simulink model "BD_PAR_SS"  (Simulink 10.3)
settings: Solver=ode1  StartTime=0.0  StopTime=max(cyc_mph(:,1))  FixedStep=1  MaxStep=1  RelTol=1e-3  AbsTol=1e-3
undefined symbols (not defined in the file): acc_elec_eff, acc_elec_pwr, acc_mech_eff, amb_tmp, cs_charge_deplete_bool, cs_electric_decel_spd, cs_electric_launch_spd_hi, cs_electric_launch_spd_lo, cs_hi_soc, cs_lo_soc, cs_off_trq_frac, cyc_avg_time, cyc_cargo_mass, cyc_elevation_init, cyc_filter_bool, cyc_grade, cyc_mph, ess_module_num, ess_on, ess_voc, ex_calc, ex_cat_co_frac, ex_cat_ext_cp, ex_cat_ext_emisv, ex_cat_ext_init_tmp, ex_cat_ext_mass, ex_cat_ext_sarea, ex_cat_hc_frac, ex_cat_i2p_th_cond, ex_cat_i2x_emisv, ex_cat_i2x_th_cond, ex_cat_int_cp, ex_cat_int_init_tmp, ex_cat_int_mass, ex_cat_int_sarea, ex_cat_lim, ex_cat_m2i_th_cond, ex_cat_m2i_tmp, ex_cat_m2p_emisv, ex_cat_mon_cp, ex_cat_mon_init_tmp, ex_cat_mon_mass, ex_cat_mon_sarea, ex_cat_monf_sarea, ex_cat_moni_sarea, ex_cat_nox_frac, ex_cat_p2x_th_cond, ex_cat_pcm_ecp, ex_cat_pcm_mass, ex_cat_pcm_tmp, ex_cat_pipe_cp, ex_cat_pipe_emisv, ex_cat_pipe_init_tmp, ex_cat_pipe_mass, ex_cat_pipe_sarea, ex_cat_pm_frac, ex_cat_tmp_range, ex_gas_cp, ex_manif_cp, ex_manif_emisv ... (+73)
libraries: lib_controls x6, lib_vehicle x3, lib_accessory x2, lib_interactive x1, lib_energy_storage x1, lib_fuel_converter x1
(part 5 of 6)

== system BD_PAR_SS/exhaust sys <ex>/ex gas heat flow/Block NOTES ==
  note: EXHAUST GAS HEAT TRANSFER
      | This block models the heat loss from the exhaust gas as it flows from the engine through the manifold,
      | downpipe, and catalytic converter.  Also included is the increase in gas temperature within the converter
      | due to the catalysis of HC, CO, and NOx. The block is conditionally executed only if engine_on=1.

== system BD_PAR_SS/exhaust sys <ex>/ex gas heat flow/converter ==
  h,exg : Inport
  Cexg : Inport  Port=2
  Texgi : Inport  Port=3
  Tex : Inport  Port=4
  " Q/C" : Product  Inputs=/*  SaturateOnIntegerOverflow=on
  1/A : Gain  Gain=1/(ex_cat_moni_sarea+ex_cat_int_sarea-ex_cat_mon_sarea)  SaturateOnIntegerOverflow=on
  Demux3 : Demux  Outputs=2
  MinMax : MinMax  Inputs=2
  Mux16 : Mux
  Qci2g_ : Fcn  Expr=u(1)*(ex_cat_int_sarea - ex_cat_mon_sarea)*(u(3)-u(4))
  Qcm2g_ : Fcn  Expr=u(1)*ex_cat_moni_sarea*(u(2)-u(4))
  Selector3 : Selector  InputPortWidth=5  IndexOptions=Index vector (dialog)  Indices=[ 1 2 ]  OutputSizes=1
  T : Sum  SaturateOnIntegerOverflow=on
  T1 : Sum  SaturateOnIntegerOverflow=on
  Texgo : Outport  OutputWhenDisabled=reset  InitialOutput=amb_tmp
  Qcm2g : Outport  Port=2  OutputWhenDisabled=reset  InitialOutput=0
  Qci2g : Outport  Port=3  OutputWhenDisabled=reset  InitialOutput=0
  wires:
  Cexg/1 -> " Q/C"/1, 1/A/1
  h,exg/1 -> MinMax/2
  1/A/1 -> MinMax/1
  MinMax/1 -> Mux16/1
  Tex/1 -> Selector3/1
  Selector3/1 -> Demux3/1
  Demux3/1 -> Mux16/2
  Demux3/2 -> Mux16/3
  Texgi/1 -> T/2, Mux16/4
  Mux16/1 -> Qcm2g_/1, Qci2g_/1
  Qci2g_/1 -> T1/2, Qci2g/1
  Qcm2g_/1 -> T1/1, Qcm2g/1
  " Q/C"/1 -> T/1
  T1/1 -> " Q/C"/2
  T/1 -> Texgo/1

== system BD_PAR_SS/exhaust sys <ex>/ex gas heat flow/inlet pipe ==
  h,exg : Inport
  Cexg : Inport  Port=2
  Texgi : Inport  Port=3
  Tex : Inport  Port=4
  " Q/C" : Product  Inputs=/*  SaturateOnIntegerOverflow=on
  A : Gain  Gain=ex_cat_pipe_sarea  SaturateOnIntegerOverflow=on
  Memory : Memory  InitialCondition=cyc_mph(1,2)*.447
  MinMax : MinMax  Inputs=2
  Mux19 : Mux  Inputs=3
  Selector2 : Selector  InputPortWidth=5  IndexOptions=Index vector (dialog)  Indices=3  OutputSizes=1
  T : Sum  SaturateOnIntegerOverflow=on
  Ts-Tex,ave : Fcn  Expr=u(2) - (u(3)+u(1))/2
  tailpipe  emis : Product  SaturateOnIntegerOverflow=on
  Texgo : Outport  OutputWhenDisabled=reset  InitialOutput=amb_tmp
  tag scope: Qp2g=global, Tgpo=global
  wires:
  h,exg/1 -> A/1
  MinMax/1 -> tailpipe  emis/1
  A/1 -> MinMax/2
  Cexg/1 -> MinMax/1, " Q/C"/1
  tailpipe  emis/1 -> " Q/C"/2, [Qp2g]
  " Q/C"/1 -> T/1
  Texgi/1 -> T/2, Mux19/1
  T/1 -> Texgo/1, [Tgpo], Memory/1
  Tex/1 -> Selector2/1
  Mux19/1 -> Ts-Tex,ave/1
  Ts-Tex,ave/1 -> tailpipe  emis/2
  Selector2/1 -> Mux19/2
  Memory/1 -> Mux19/3

== system BD_PAR_SS/exhaust sys <ex>/ex gas heat flow/manifold  ==
  h,exg : Inport
  Cexg : Inport  Port=2
  Texgi : Inport  Port=3
  Tex : Inport  Port=4
  " Q/C" : Product  Inputs=/*  SaturateOnIntegerOverflow=on
  A : Gain  Gain=ex_manif_sarea  SaturateOnIntegerOverflow=on
  Memory : Memory  InitialCondition=cyc_mph(1,2)*.447
  MinMax : MinMax  Inputs=2
  Mux19 : Mux  Inputs=3
  Selector1 : Selector  InputPortWidth=5  IndexOptions=Index vector (dialog)  Indices=5  OutputSizes=1
  T : Sum  SaturateOnIntegerOverflow=on
  Ts-Tex,ave : Fcn  Expr=u(2) - (u(3)+u(1))/2
  tailpipe  emis : Product  SaturateOnIntegerOverflow=on
  Texgo : Outport  OutputWhenDisabled=reset  InitialOutput=amb_tmp
  tag scope: Qma2g=global, Tgmo=global
  wires:
  h,exg/1 -> A/1
  MinMax/1 -> tailpipe  emis/1
  A/1 -> MinMax/2
  Cexg/1 -> MinMax/1, " Q/C"/1
  " Q/C"/1 -> T/1
  T/1 -> [Tgmo], Texgo/1, Memory/1
  tailpipe  emis/1 -> " Q/C"/2, [Qma2g]
  Tex/1 -> Selector1/1
  Selector1/1 -> Mux19/2
  Mux19/1 -> Ts-Tex,ave/1
  Memory/1 -> Mux19/3
  Ts-Tex,ave/1 -> tailpipe  emis/2
  Texgi/1 -> Mux19/1, T/2

== system BD_PAR_SS/exhaust sys <ex>/ex sys heat flow/Block NOTES ==
  note: CATALYTIC CONVERTER HEAT LOSS
      | This block models the heat loss from a catalytic converter (conventional or vacuum-insulated).
      | Convection (as a function of vehicle speed), radiation, and conduction effects are included.
      | Converter monolith (m), interior (i), pipe (p), and exterior (x) and engine manifold
      | heat flows are estimated based on the temperatures from the previous iteration.

== system BD_PAR_SS/exhaust sys <ex>/removal efficiencies/removal efficiencies (base ADVISOR) ==
  Ex Cat T (C) : Inport
  Enable : EnablePort  StatesWhenEnabling=reset
  CO temp eff : Lookup  InputValues=ex_cat_tmp_range  Table=ex_cat_co_frac  SaturateOnIntegerOverflow=on
  HC temp eff : Lookup  InputValues=ex_cat_tmp_range  Table=ex_cat_hc_frac  SaturateOnIntegerOverflow=on
  Mux : Mux
  NOx temp eff : Lookup  InputValues=ex_cat_tmp_range  Table=ex_cat_nox_frac  SaturateOnIntegerOverflow=on
  PM temp eff : Lookup  InputValues=ex_cat_tmp_range  Table=ex_cat_pm_frac  SaturateOnIntegerOverflow=on
  removal effs : Outport  OutputWhenDisabled=reset  InitialOutput=0
  wires:
  Ex Cat T (C)/1 -> PM temp eff/1, NOx temp eff/1, CO temp eff/1, HC temp eff/1
  Mux/1 -> removal effs/1
  PM temp eff/1 -> Mux/4
  NOx temp eff/1 -> Mux/3
  HC temp eff/1 -> Mux/1
  CO temp eff/1 -> Mux/2

== system BD_PAR_SS/exhaust sys <ex>/removal efficiencies/removal efficiencies ORNL ==
  gas_flow (g/s) : Inport
  Ex Gas T (C) : Inport  Port=2
  O2_exh (g/s) : Inport  Port=3
  emis Engine Out (g/s) : Inport  Port=4
  Ex Cat T (C) : Inport  Port=5
  Enable : EnablePort  StatesWhenEnabling=reset
  CO : Terminator
  CO-Conversion : Subsystem
  Constant : Constant  Value=1200
  Demux : Demux
  HC-Conversion : Subsystem
  Mux : Mux
  NOx_Eff : Subsystem
  PM : Terminator
  PM temp eff : Lookup  InputValues=ex_cat_tmp_range  Table=ex_cat_pm_frac  SaturateOnIntegerOverflow=on
  Product : Product  Inputs=/*  SaturateOnIntegerOverflow=on
  Volume  Flow (m^3/sec) : Gain  Gain=2.96E6  SaturateOnIntegerOverflow=on
  removal effs : Outport  OutputWhenDisabled=reset  InitialOutput=0
  wires:
  Mux/1 -> removal effs/1
  gas_flow (g/s)/1 -> CO-Conversion/4(ex_gas_flow), HC-Conversion/4(ex_gas_flow), Product/2
  Ex Cat T (C)/1 -> PM temp eff/1
  O2_exh (g/s)/1 -> CO-Conversion/3(O2_exh), HC-Conversion/3(O2_exh)
  CO-Conversion/1(CO_eff) -> Mux/2
  HC-Conversion/1(HC_eff) -> Mux/1
  NOx_Eff/1(NOx_eff) -> Mux/3
  PM temp eff/1 -> Mux/4
  Ex Gas T (C)/1 -> NOx_Eff/2(Ex_temp), CO-Conversion/2(T_exh), HC-Conversion/2(T_exh)
  Volume  Flow (m^3/sec)/1 -> NOx_Eff/1(vol_flow), CO-Conversion/1(vol_flow), HC-Conversion/1(vol_flow)
  Demux/1 -> NOx_Eff/3(HC_Inlet)
  Demux/3 -> NOx_Eff/4(NOx_Inlet)
  Demux/2 -> CO/1
  Demux/4 -> PM/1
  emis Engine Out (g/s)/1 -> Demux/1
  Constant/1 -> Product/1
  Product/1 -> Volume  Flow (m^3/sec)/1

== system BD_PAR_SS/fuel converter  <fc>/engine speed estimator/Block NOTES ==
  note: If the clutch is engaged and the trace was missed in the previous time step:
      | The estimated engine speed for the current time step is the actual engine
      | speed from the previous time step.
      |
      | If the clutch is disengaged and the speed is commanded to increase (spin up):
      | The engine speed is the lesser of the commanded speed and the maximum
      | speed attainable given the engine capability.
      |
      | If the clutch is disengaged at the speed is commanded to decrease (spin down):
      | The engine speed is computed by integrating with respect to time the ratio of
      |  closed-throttle torque to engine inertia.
      |
      | Otherwise:
      | The engine speed is equal to the speed command, but no greater than the
      | engine's maximum speed nor less than the engine's idle speed (if the engine is on.)

== system BD_PAR_SS/fuel converter  <fc>/engine speed estimator/dt ==
  Clock : Clock
  Memory1 : Memory  InitialCondition=-0.1
  Sum1 : Sum  Inputs=+-  InputSameDT=on  SaturateOnIntegerOverflow=on  OutDataTypeStr=Inherit: Same as first input
  out_1 : Outport  InitialOutput=0
  wires:
  Sum1/1 -> out_1/1
  Memory1/1 -> Sum1/2
  Clock/1 -> Memory1/1, Sum1/1

== system BD_PAR_SS/fuel converter  <fc>/engine speed estimator/effect of inertia (Nm) ==
  req'd spd (rad/s) : Inport
  prev spd : Inport  Port=2
  Clock : Clock
  Constant : Constant  Value=fc_inertia
  Memory : Memory  InitialCondition=-0.1
  Product1 : Product  Inputs=**/  InputSameDT=on  RndMeth=Zero  SaturateOnIntegerOverflow=on  OutDataTypeStr=Inherit: Same as first input
  Sum : Sum  Inputs=+-  InputSameDT=on  SaturateOnIntegerOverflow=on  OutDataTypeStr=Inherit: Same as first input
  Sum1 : Sum  Inputs=+-  InputSameDT=on  SaturateOnIntegerOverflow=on  OutDataTypeStr=Inherit: Same as first input
  (Nm) : Outport  InitialOutput=0
  wires:
  Constant/1 -> Product1/1
  Clock/1 -> Sum1/1, Memory/1
  Memory/1 -> Sum1/2
  Product1/1 -> (Nm)/1
  prev spd/1 -> Sum/2
  req'd spd (rad/s)/1 -> Sum/1
  Sum1/1 -> Product1/3
  Sum/1 -> Product1/2

== system BD_PAR_SS/fuel converter  <fc>/engine speed estimator/just started spin-down/spin-up ==
  state : Inport
  Logical Operator : Logic
  Logical Operator1 : Logic  Operator=NOT  Inputs=1
  Memory1 : Memory  InitialCondition=1
  trigger : Outport  InitialOutput=0
  wires:
  state/1 -> Memory1/1, Logical Operator/1
  Logical Operator/1 -> trigger/1
  Logical Operator1/1 -> Logical Operator/2
  Memory1/1 -> Logical Operator1/1

== system BD_PAR_SS/fuel converter  <fc>/engine speed estimator/no-lag Reset Integrator ==
  in_1 : Inport
  in_2 : Inport  Port=2
  in_3 : Inport  Port=3
  Constant : Constant  Value=0
  Memory : Memory  InitialCondition=initval
  Product : Product  InputSameDT=on  RndMeth=Zero  SaturateOnIntegerOverflow=on  OutDataTypeStr=Inherit: Same as first input
  Sum : Sum  InputSameDT=on  SaturateOnIntegerOverflow=on  OutDataTypeStr=Inherit: Same as first input
  Switch : Switch  Threshold=eps  SaturateOnIntegerOverflow=on  InputSameDT=on
  dt : Subsystem
  in_2==0 : RelationalOperator  Operator===  RndMeth=Nearest  InputSameDT=on
  out_1 : Outport  InitialOutput=0
  wires:
  Constant/1 -> in_2==0/2
  in_2==0/1 -> Switch/2
  Switch/1 -> Memory/1, out_1/1
  Sum/1 -> Switch/1
  Memory/1 -> Sum/1
  Product/1 -> Sum/2
  dt/1(out_1) -> Product/1
  in_1/1 -> Product/2
  in_2/1 -> in_2==0/1
  in_3/1 -> Switch/3

== system BD_PAR_SS/fuel converter  <fc>/engine torque/Block NOTES ==
  note: If the engine is not spinning down with the clutch disengaged:
      | 1.  Engine brake (aka map) torque is given by the required shaft
      | torque plus enough torque to accelerate the engine's rotating
      | parts as commanded and torque to power the accessories,
      | subject to the engine's torque limits at the current speed.
      | 2.  Shaft torque is engine brake torque less the effects of inertia
      | and accessories.
      |
      | If the engine is spinning down:
      | 1.  Engine brake/map torque is the closed-throttle torque.
      | 2.  Shaft torque is zero.

== system BD_PAR_SS/fuel converter  <fc>/engine torque/T_closed throttle ==
  w_APU : Inport
  Saturation : Saturate  UpperLimit=max(fc_map_spd)*fc_spd_scale  LowerLimit=min(fc_map_spd)*fc_spd_scale
  ctt lookup : Lookup  InputValues=fc_map_spd*fc_spd_scale  Table=fc_ct_trq*fc_trq_scale  SaturateOnIntegerOverflow=on
  T_closed throttle : Outport  InitialOutput=0
  wires:
  w_APU/1 -> Saturation/1
  Saturation/1 -> ctt lookup/1
  ctt lookup/1 -> T_closed throttle/1

== system BD_PAR_SS/fuel converter  <fc>/engine torque/T_max ==
  w_APU : Inport
  Saturation1 : Saturate  UpperLimit=max(fc_map_spd)*fc_spd_scale  LowerLimit=min(fc_map_spd)*fc_spd_scale
  max_torque lookup : Lookup  InputValues=fc_map_spd*fc_spd_scale  Table=fc_max_trq*fc_trq_scale  SaturateOnIntegerOverflow=on
  T_max : Outport  InitialOutput=0
  tag scope: engine_rpm=global
  wires:
  Saturation1/1 -> [engine_rpm], max_torque lookup/1
  max_torque lookup/1 -> T_max/1
  w_APU/1 -> Saturation1/1

== system BD_PAR_SS/fuel converter  <fc>/engine torque/effect of inertia (Nm) ==
  engine spd (rad/s) : Inport
  >=0 : Saturate  UpperLimit=inf  LowerLimit=0
  Block NOTES : Subsystem
      mask Display: disp('Block\nNOTES')
  Clock : Clock
  Constant : Constant  Value=fc_inertia
  Constant1 : Constant  Value=max(fc_max_trq)*fc_trq_scale
  Constant2 : Constant  Value=0.01
  Memory : Memory  InitialCondition=-0.1
  Memory1 : Memory  InitialCondition=vc_idle_spd*vc_key_on(1,2)
  Memory2 : Memory
  MinMax : MinMax  Inputs=2  InputSameDT=on  SaturateOnIntegerOverflow=on
  Product : Product  InputSameDT=on  RndMeth=Zero  SaturateOnIntegerOverflow=on  OutDataTypeStr=Inherit: Same as first input
  Product1 : Product  Inputs=*/*  InputSameDT=on  RndMeth=Zero  SaturateOnIntegerOverflow=on  OutDataTypeStr=Inherit: Same as first input
  Relational : RelationalOperator  Operator=>  RndMeth=Nearest  InputSameDT=on
  Sum : Sum  Inputs=+-  InputSameDT=on  SaturateOnIntegerOverflow=on  OutDataTypeStr=Inherit: Same as first input
  Sum1 : Sum  Inputs=+-  InputSameDT=on  SaturateOnIntegerOverflow=on  OutDataTypeStr=Inherit: Same as first input
  Sum2 : Sum  Inputs=-+  InputSameDT=on  SaturateOnIntegerOverflow=on  OutDataTypeStr=Inherit: Same as first input
  Switch : Switch  Threshold=eps  SaturateOnIntegerOverflow=on  InputSameDT=on
  engine inertia as a function of total vehicle inertia (generous approximation) : Subsystem
  (Nm) : Outport  InitialOutput=0
  wires:
  engine spd (rad/s)/1 -> Sum/1, Memory1/1
  Constant2/1 -> Relational/2
  Sum2/1 -> Relational/1
  >=0/1 -> Switch/1
  Relational/1 -> Memory2/1
  Memory2/1 -> Switch/2
  Clock/1 -> Sum1/1, Memory/1
  Memory/1 -> Sum1/2
  Constant/1 -> Product1/3
  Sum1/1 -> Product1/2
  Switch/1 -> Product1/1
  [mpha] -> Sum2/1
  [cyc_mph_r] -> Sum2/2
  MinMax/1 -> (Nm)/1
  Product1/1 -> MinMax/2
  engine inertia as a function of total vehicle inertia (generous approximation)/1(Out1) -> Product/1
  Constant1/1 -> Product/2
  Product/1 -> MinMax/1
  Memory1/1 -> Sum/2
  Sum/1 -> Switch/3, >=0/1

== system BD_PAR_SS/gearbox <gb>/Pout/Pin, neglecting inertia/Pout/Pin (neglecting inertia) ==
  in_1 : Inport
  in_2 : Inport  Port=2
  Fcn : Fcn  Expr=1/u
  Product : Product  SaturateOnIntegerOverflow=on
  out_1 : Outport  InitialOutput=0
  wires:
  in_1/1 -> Product/1
  Fcn/1 -> Product/2
  Product/1 -> out_1/1
  in_2/1 -> Fcn/1

== system BD_PAR_SS/gearbox <gb>/Pout/Pin, neglecting inertia/make division bombproof ==
  note: only add eps if Tin-Tinertia is == 0 (this avoids problems when Tin-Tineratia == -eps
      | which happens from time to time
  Tin-Tinertia : Inport
  Block NOTES : Subsystem
      mask Display: disp('Block\nNOTES')
  Constant : Constant  Value=eps
  Constant1 : Constant  Value=0
  Product : Product  SaturateOnIntegerOverflow=on
  Relational Operator1 : RelationalOperator  Operator===  RndMeth=Nearest  InputSameDT=on
  make division bombproof : Sum  SaturateOnIntegerOverflow=on
  Out1 : Outport
  wires:
  Tin-Tinertia/1 -> make division bombproof/1, Relational Operator1/1
  Constant1/1 -> Relational Operator1/2
  Product/1 -> make division bombproof/2
  Relational Operator1/1 -> Product/1
  Constant/1 -> Product/2
  make division bombproof/1 -> Out1/1

== system BD_PAR_SS/gearbox <gb>/loss (Nm)/3D discrete lookup table (sfun) ==
  lookup speed (rad/s) : Inport
  lookup trq (Nm) : Inport  Port=2
  "gear_number  (e.g., 1, 2, 3)" : Inport  Port=3
  Mux : Mux  Inputs=3
  Saturation : Saturate  UpperLimit=max(tx_map_spd)  LowerLimit=min(tx_map_spd)
  Saturation1 : Saturate  UpperLimit=max(tx_map_trq)  LowerLimit=min(tx_map_trq)
  Saturation2 : Saturate  UpperLimit=size(tx_eff_map,3)  LowerLimit=1
  discrete interp2d : S-Function  FunctionName=sfun_discreteLookup3d  Parameters=tx_map_trq, tx_map_spd, tx_eff_map  SFunctionDeploymentMode=off  EnableBusSupport=off
  tx_eff : Outport
  wires:
  discrete interp2d/1 -> tx_eff/1
  Mux/1 -> discrete interp2d/1
  lookup speed (rad/s)/1 -> Saturation/1
  Saturation/1 -> Mux/1
  lookup trq (Nm)/1 -> Saturation1/1
  Saturation1/1 -> Mux/2
  "gear_number  (e.g., 1, 2, 3)"/1 -> Saturation2/1
  Saturation2/1 -> Mux/3

== system BD_PAR_SS/gearbox <gb>/loss (Nm)/Block NOTES ==
  note: 09/20/02:tm modifed lower input to switch after T_loss_at_input to pass the
      | total torque input as the loss when tx_eff=0
      | 5 July 2001:mpo changing loss block to a lookup table methodology
      | 12/20/00:tm revised loss saturation block. lower limit changed
      | from 1 to 0 and upper limit changed from 100 to inf to prevent over or under penalties
  note: Revision Notes:

== system BD_PAR_SS/mechanical accessory loads <acc>/Mechanical Accessory Loads v2 <acc>/Accessory SDO ==
  data bus : Inport
  Demux : Demux  Outputs=6
      settings: DisplayOption=none
  To Workspace : ToWorkspace  VariableName=acc_mech_trq_r  SampleTime=-1
  To Workspace1 : ToWorkspace  VariableName=acc_mech_pwr_a  SampleTime=-1
  To Workspace2 : ToWorkspace  VariableName=acc_mech_trq_est  SampleTime=-1
  To Workspace3 : ToWorkspace  VariableName=acc_mech_pwr_r  SampleTime=-1
  To Workspace4 : ToWorkspace  VariableName=acc_mech_trq_a  SampleTime=-1
  To Workspace5 : ToWorkspace  VariableName=acc_mech_pwr_est  SampleTime=-1
  mechanical power logging : Subsystem  mask{eff=acc_mech_eff}
      mask prompts: eff "efficiency of accessory systems (decimal)"
  wires:
  Demux/6 -> To Workspace5/1
  Demux/5 -> To Workspace2/1
  Demux/3 -> To Workspace4/1
  Demux/2 -> To Workspace3/1
  Demux/1 -> To Workspace/1
  Demux/4 -> To Workspace1/1, mechanical power logging/1(In1)
  data bus/1 -> Demux/1

== system BD_PAR_SS/mechanical accessory loads <acc>/Mechanical Accessory Loads v2 <acc>/Block NOTES ==
  note: In this model, only one speed is used to predict accessory
      | loading. The forward model is "dummied" out.
  note: A third input is given for accessory load speed. This is done so that
      | the accessory block can use fc_spd_est which is an estimated vehicle speed
      | (equal to fc_spd_out under normal circumstances).
      | Using fc_spd_est provides total compatibility with ADVISOR v3.2
  note: In terms of an interface, the model assumes belt-driven mechanical loads
      | that run off of a prime mover shaft (e.g., engine shaft)
      |
      | This model takes in requested driveline torque and speed requests and
      | augments torque due to belt driven accessories.
      |
      | The torque passed along down to the driveline is only torque to move the
      | vehicle.
  note: This is the mechanical auxiliary loads model.

== system BD_PAR_SS/mechanical accessory loads <acc>/Mechanical Accessory Loads v2 <acc>/backward model ==
  note: Power, W, input to accessory
  note: T, Nm, shaft out
  note: T, Nm, driveline
  note: T, Nm, accessory
  note: w_apu, rad/s
  trq_in : Inport
  spd_in : Inport  Port=2
  acc on/off : Inport  Port=3
  Product : Product  Inputs=**  InputSameDT=on  RndMeth=Zero  SaturateOnIntegerOverflow=on  OutDataTypeStr=Inherit: Same as first input
  Product1 : Product  Inputs=**  InputSameDT=on  RndMeth=Zero  SaturateOnIntegerOverflow=on  OutDataTypeStr=Inherit: Same as first input
  Sum : Sum  Inputs=|++  InputSameDT=on  SaturateOnIntegerOverflow=on  OutDataTypeStr=Inherit: Same as first input
  acc_mech_var_loads : ToWorkspace  VariableName=acc_mech_var_load  SaveFormat=Structure  SampleTime=-1
  mechanical accessories (Nm) : Subsystem  BlockChoice=Mechanical Accessories: Const Mech Var Elect
      settings: AttributesFormatString=%<BlockChoice>  TemplateBlock=lib_accessory/mechanical accessories (Nm)  MemberBlocks=Mechanical Accessories: Const Mech Var Elect,Mechanical Accessories: Constant Mechanical & Electrical,Mechanical Accessories: Speed Dependant and Variable Electrical,Saber Dual Voltage Cosim,Saber Single Voltage Cosim,SindaTransAC
      mask Display: image(imread('bdi_acc_pic_cs.bmp'))
  trq_out : Outport
  acc_mech_trq_r : Outport  Port=2
  acc_mech_pwr_r : Outport  Port=3
  wires:
  mechanical accessories (Nm)/3(probes) -> acc_mech_var_loads/1
  [acc_on] -> Product1/2
  [acc_on] -> Product/1
  acc on/off/1 -> [acc_on]
  mechanical accessories (Nm)/2(P_mech_acc) -> Product1/1
  Product1/1 -> acc_mech_pwr_r/1
  mechanical accessories (Nm)/1(T_acc) -> Product/2
  Product/1 -> Sum/2, acc_mech_trq_r/1
  Sum/1 -> trq_out/1
  trq_in/1 -> Sum/1
  spd_in/1 -> mechanical accessories (Nm)/1(w_APU)

== system BD_PAR_SS/mechanical accessory loads <acc>/Mechanical Accessory Loads v2 <acc>/forward model ==
  note: acc torque, Nm
  note: NOTES
  note: This simplistic model may not correctly account for accessory torque and/or power
      | when the upstream torque provider is torque or speed limited
  note: Power, W, input to accessory
  note: T, Nm, shaft out
  note: driveline and
      | acc torque, Nm
  note: T, Nm, accessory
  note: acc speed, rad/s
  trq_in : Inport
  spd_in : Inport  Port=2
  acc_trq_req : Inport  Port=3
  Product1 : Product  Inputs=**  InputSameDT=on  RndMeth=Zero  SaturateOnIntegerOverflow=on  OutDataTypeStr=Inherit: Same as first input
  Sum : Sum  Inputs=|+-  InputSameDT=on  SaturateOnIntegerOverflow=on  OutDataTypeStr=Inherit: Same as first input
  trq_out : Outport
  acc_mech_trq_a : Outport  Port=2
  acc_mech_pwr_a : Outport  Port=3
  wires:
  [pm_trq_a] -> Sum/1
  acc_trq_req/1 -> [acc_trq_r]
  trq_in/1 -> [pm_trq_a]
  [acc_spd] -> Product1/2
  [acc_trq_r] -> Product1/1, Sum/2, acc_mech_trq_a/1
  Product1/1 -> acc_mech_pwr_a/1
  Sum/1 -> trq_out/1
  spd_in/1 -> [acc_spd]

== system BD_PAR_SS/motor/ controller <mc> par/N-m drive torque per W input/Block NOTES ==
  note: This block determines the ratio of req'd rotor torque to req'd electrical input power,
      |  which is proportional to efficiency if the motor is providing torque.  This ratio is used
      | to compute actual rotor torque given some input power which may be different from
      | the req'd value.
      |
      | If the denominator, the req'd input power, is zero, this block outputs inf,
      | which is a flag used by the block .../rotor drive torque available (Nm).

== system BD_PAR_SS/motor/ controller <mc> par/effect of inertia (Nm)/Block NOTES ==
  note: Torque required to accelerate the motor's inertia is calculated from the rate of change
      | of mc_spd_out_a.  It is no greater than the product of the maximum motor torque and
      | the fractional contribution of the motor's inertia to the total vehicle inertia.

== system BD_PAR_SS/motor/ controller <mc> par/effect of inertia (Nm)/motor inertia as a function of total vehicle inertia (generous approximation) ==
  gear ratio : Inport
  Product : Product  Inputs=*/  SaturateOnIntegerOverflow=on
  Sum : Sum  Inputs=++|  SaturateOnIntegerOverflow=on
  engine inertia as a fraction of total vehicle inertia  (generous approximation)--denomenator : Fcn  Expr=mc_inertia*u^2
  engine inertia as a fraction of total vehicle inertia  (generous approximation)--numerator : Fcn  Expr=mc_inertia*u^2
  veh mass calc : Subsystem
  Out1 : Outport
  wires:
  Sum/1 -> Product/2
  engine inertia as a fraction of total vehicle inertia  (generous approximation)--denomenator/1 -> Sum/2
  veh mass calc/1(Out1) -> Sum/1
  gear ratio/1 -> engine inertia as a fraction of total vehicle inertia  (generous approximation)--denomenator/1, engine inertia as a fraction of total vehicle inertia  (generous approximation)--numerator/1
  Product/1 -> Out1/1
  engine inertia as a fraction of total vehicle inertia  (generous approximation)--numerator/1 -> Product/1

== system BD_PAR_SS/motor/ controller <mc> par/enforce torque limit/Block NOTES ==
  note: This block enforces the maximum torque production and absorption
      | capability limits of the motor.  It assumes that exactly as much torque
      | can be absorbed as can be produced at a given speed.

== system BD_PAR_SS/motor/ controller <mc> par/mc tmp/Block NOTES ==
  note: This block models the thermal behavior of a motor
      | and controller  with active fluid cooling.
      | The module is modeled as a single lumped thermal mass.
      | The fan is on whenever the battery temp is > the set temp.

== system BD_PAR_SS/motor/ controller <mc> par/mc tmp/mc coolant ==
  Tcl : Inport
  "Qmc " : Inport  Port=2
  Enable : EnablePort  StatesWhenEnabling=reset
  Constant : Constant  Value=mc_tstat
  Product1 : Product  SaturateOnIntegerOverflow=on
  Relational Operator : RelationalOperator  Operator=<=  RndMeth=Nearest  InputSameDT=on
  Qmc_clt : Outport  OutputWhenDisabled=reset  InitialOutput=0
  wires:
  Tcl/1 -> Relational Operator/2
  Constant/1 -> Relational Operator/1
  "Qmc "/1 -> Product1/2
  Product1/1 -> Qmc_clt/1
  Relational Operator/1 -> Product1/1

== system BD_PAR_SS/motor/ controller <mc> par/motor speed estimator/Block NOTES ==
  note: The requested motor speed is replaced by an estimate of the
      | motor's previous speed, for loss and max. torque calculations,
      | whenever the vehicle missed the trace by more than 1 mph
      | on the last time step.

== system BD_PAR_SS/motor/ controller <mc> par/rotor drive torque available (Nm)/Block NOTES ==
  note: This block computes the actual rotor torque given the actual motor input power and
      | the ratio (req'd rotor torque)/(req'd input power).
      |
      | If the above ratio has the value inf, which implies that the req'd input power is zero,
      | then the actual rotor torque is assumed to be zero.  This is not reflective of reality, of course:
      | with zero input power, the rotor torque would be the motor spin-loss torque at the given speed.
      | Because this simplification occurs only when req'd input power is zero, it does not.
      | affect fuel economy or max effort acceleration calculations.

== system BD_PAR_SS/vehicle <veh>/force req'd to accelerate (N)/current veh mass ==
  Constant3 : Constant  Value=veh_mass
  Sum1 : Sum  Inputs=|++  SaturateOnIntegerOverflow=on
  Out1 : Outport
  wires:
  Constant3/1 -> Sum1/1
  [veh_cargo_mass] -> Sum1/2
  Sum1/1 -> Out1/1

== system BD_PAR_SS/vehicle <veh>/force req'd to ascend (N)/current veh mass ==
  Constant3 : Constant  Value=veh_mass
  Sum1 : Sum  Inputs=|++  SaturateOnIntegerOverflow=on
  Out1 : Outport
  wires:
  Constant3/1 -> Sum1/1
  [veh_cargo_mass] -> Sum1/2
  Sum1/1 -> Out1/1

== system BD_PAR_SS/vehicle <veh>/record achieved force outputs/force req'd to accelerate (N)1 ==
  v(m/s) : Inport
  v prev : Inport  Port=2
  Clock : Clock
  Memory : Memory  InitialCondition=-0.1
  Product1 : Product  Inputs=**/  SaturateOnIntegerOverflow=on
  Sum : Sum  Inputs=+-  SaturateOnIntegerOverflow=on
  Sum1 : Sum  Inputs=+-  SaturateOnIntegerOverflow=on
  current veh mass : Subsystem
  (N) : Outport  InitialOutput=0
  wires:
  current veh mass/1(Out1) -> Product1/1
  Clock/1 -> Sum1/1, Memory/1
  Memory/1 -> Sum1/2
  Product1/1 -> (N)/1
  v prev/1 -> Sum/2
  v(m/s)/1 -> Sum/1
  Sum1/1 -> Product1/3
  Sum/1 -> Product1/2

== system BD_PAR_SS/vehicle <veh>/record achieved force outputs/force req'd to ascend (N)1 ==
  average vehicle speed over time step (m/s) : Inport
  Constant : Constant  Value=veh_gravity
  Constant1 : Constant  Value=0
  Product : Product  Inputs=3  SaturateOnIntegerOverflow=on
  Switch : Switch  SaturateOnIntegerOverflow=on  InputSameDT=on
  Trigonometric Function : Trigonometry  Operator=atan
  Trigonometric Function1 : Trigonometry
  current veh mass : Subsystem
  (N) : Outport  InitialOutput=0
  wires:
  current veh mass/1(Out1) -> Product/3
  average vehicle speed over time step (m/s)/1 -> Switch/2
  Constant1/1 -> Switch/3
  Switch/1 -> (N)/1
  Product/1 -> Switch/1
  Constant/1 -> Product/1
  [grade] -> Trigonometric Function/1
  Trigonometric Function1/1 -> Product/2
  Trigonometric Function/1 -> Trigonometric Function1/1

== system BD_PAR_SS/vehicle <veh>/record achieved force outputs/force req'd to overcome aerodynamic drag (N)1 ==
  average vehicle speed over time step (m/s) : Inport
  Constant : Constant  Value=veh_air_density*veh_CD*veh_FA*0.5
  Product : Product  Inputs=3  SaturateOnIntegerOverflow=on
  D aero(N) : Outport  InitialOutput=0
  wires:
  Product/1 -> D aero(N)/1
  Constant/1 -> Product/3
  average vehicle speed over time step (m/s)/1 -> Product/2, Product/1

== system BD_PAR_SS/vehicle <veh>/record achieved force outputs/rolling resistance force ==
  average vehicle speed over time step (m/s) : Inport
  force req'd to overcome rolling resistance (N) : lib_vehicle/Submodels/force req'd to overcome rolling resistance (N)  SystemSampleTime=-1  VariantActivationTime=update diagram  Latency=0  AutoFrameSizeCalculation=off
  Fr (N) : Outport
  wires:
  average vehicle speed over time step (m/s)/1 -> force req'd to overcome rolling resistance (N)/1
  force req'd to overcome rolling resistance (N)/1 -> Fr (N)/1

== system BD_PAR_SS/wheel and axle  front/rear <wh>/front force/brake request  controller interface ==
  F_front_brake_req : Outport  InitialOutput=0
  wires:
  [F_front_brake_req] -> F_front_brake_req/1

== system BD_PAR_SS/wheel and axle  front/rear <wh>/loss (Nm)/veh mass calc ==
  Constant : Constant  Value=veh_mass
  Sum : Sum  Inputs=|++  SaturateOnIntegerOverflow=on
  Out1 : Outport
  wires:
  Sum/1 -> Out1/1
  Constant/1 -> Sum/2
  [veh_cargo_mass] -> Sum/1

== system BD_PAR_SS/wheel and axle  front/rear <wh>/rear force/brake request controller interface1 ==
  F_rear_brake_req : Outport  InitialOutput=0
  wires:
  [F_rear_brake_req] -> F_rear_brake_req/1

== system BD_PAR_SS/wheel and axle  front/rear <wh>/tire slip model (m/s)/Block NOTES ==
  note: This block implements the effects of finite tire slip (with respect to the road) on the
      | vehicle speed/wheel speed relationship.  Slip is defined as s=(omega*r - v) / v.  The
      | one-to-one mapping of slip to normalized tractive force, F_tract/W_front_axle, up to
      | the maximum, is stored in the variables "wh_slip" and "wh_slip_force_coeff."  The
      | slip calculation here is overridden if the actual axle speed and the requested axle
      | speed are the same, indicating that no drivetrain speed limits were encountered.

== system BD_PAR_SS/wheel and axle  front/rear <wh>/tire slip model (m/s)/front axle ==
  In1 : Inport
  In2 : Inport  Port=2
  Abs : Abs  SaturateOnIntegerOverflow=on
  Constant3 : Constant  Value=0
  F/W : Product  Inputs=*/  SaturateOnIntegerOverflow=on
  Product : Product  SaturateOnIntegerOverflow=on
  Relational Operator : RelationalOperator  Operator=~=  RndMeth=Nearest  InputSameDT=on
  Saturation : Saturate  UpperLimit=max(wh_slip_force_coeff)  LowerLimit=min(wh_slip_force_coeff)
  Sign : Signum
  Switch : Switch  SaturateOnIntegerOverflow=on  InputSameDT=on
  s=s(F/W) : Lookup  InputValues=wh_slip_force_coeff  Table=wh_slip  SaturateOnIntegerOverflow=on
  Out1 : Outport
  wires:
  Product/1 -> Out1/1
  In1/1 -> F/W/2
  In2/1 -> Sign/1, Abs/1
  s=s(F/W)/1 -> Product/1
  Sign/1 -> Product/2
  F/W/1 -> Switch/1
  Switch/1 -> Saturation/1
  Saturation/1 -> s=s(F/W)/1
  Abs/1 -> Relational Operator/1, F/W/1
  Relational Operator/1 -> Switch/2
  Constant3/1 -> Relational Operator/2, Switch/3

== system BD_PAR_SS/wheel and axle  front/rear <wh>/tire slip model (m/s)/rear axle ==
  In1 : Inport
  In2 : Inport  Port=2
  Abs : Abs  SaturateOnIntegerOverflow=on
  Constant3 : Constant  Value=0
  F/W : Product  Inputs=*/  SaturateOnIntegerOverflow=on
  Product : Product  SaturateOnIntegerOverflow=on
  Relational Operator : RelationalOperator  Operator=~=  RndMeth=Nearest  InputSameDT=on
  Saturation : Saturate  UpperLimit=max(wh_slip_force_coeff)  LowerLimit=min(wh_slip_force_coeff)
  Sign : Signum
  Switch : Switch  SaturateOnIntegerOverflow=on  InputSameDT=on
  s=s(F/W) : Lookup  InputValues=wh_slip_force_coeff  Table=wh_slip  SaturateOnIntegerOverflow=on
  Out1 : Outport
  wires:
  Product/1 -> Out1/1
  In1/1 -> F/W/2
  In2/1 -> Sign/1, Abs/1
  s=s(F/W)/1 -> Product/1
  Sign/1 -> Product/2
  F/W/1 -> Switch/1
  Switch/1 -> Saturation/1
  Saturation/1 -> s=s(F/W)/1
  Abs/1 -> Relational Operator/1, F/W/1
  Relational Operator/1 -> Switch/2
  Constant3/1 -> Relational Operator/2, Switch/3

== system BD_PAR_SS/wheel and axle  front/rear <wh>/tire slip model (rad/s)/front slip ==
  In1 : Inport
  In2 : Inport  Port=2
  Abs : Abs  SaturateOnIntegerOverflow=on
  F/W : Product  Inputs=*/  SaturateOnIntegerOverflow=on
  Product : Product  SaturateOnIntegerOverflow=on
  Saturation : Saturate  UpperLimit=max(wh_slip_force_coeff)  LowerLimit=min(wh_slip_force_coeff)
  Sign : Signum
  s=s(F/W) : Lookup  InputValues=wh_slip_force_coeff  Table=wh_slip  SaturateOnIntegerOverflow=on
  Out1 : Outport
  wires:
  Product/1 -> Out1/1
  In1/1 -> F/W/2
  s=s(F/W)/1 -> Product/1
  In2/1 -> Sign/1, Abs/1
  Sign/1 -> Product/2
  Abs/1 -> F/W/1
  F/W/1 -> Saturation/1
  Saturation/1 -> s=s(F/W)/1

== system BD_PAR_SS/wheel and axle  front/rear <wh>/tire slip model (rad/s)/rear slip ==
  In1 : Inport
  In2 : Inport  Port=2
  Abs : Abs  SaturateOnIntegerOverflow=on
  F/W : Product  Inputs=*/  SaturateOnIntegerOverflow=on
  Product : Product  SaturateOnIntegerOverflow=on
  Saturation : Saturate  UpperLimit=max(wh_slip_force_coeff)  LowerLimit=min(wh_slip_force_coeff)
  Sign : Signum
  s=s(F/W) : Lookup  InputValues=wh_slip_force_coeff  Table=wh_slip  SaturateOnIntegerOverflow=on
  Out1 : Outport
  wires:
  Product/1 -> Out1/1
  In1/1 -> F/W/2
  s=s(F/W)/1 -> Product/1
  In2/1 -> Sign/1, Abs/1
  Sign/1 -> Product/2
  Abs/1 -> F/W/1
  F/W/1 -> Saturation/1
  Saturation/1 -> s=s(F/W)/1

== system BD_PAR_SS/<vc> par/parallel clutch control/gearbox speed estimator/Block NOTES ==
  note: The requested engine speed is replaced by an estimate of the
      | engine's previous speed whenever the vehicle missed the trace
      |  by more than 1 mph on the last time step.

== system BD_PAR_SS/<vc> par/parallel clutch control/gearbox speed estimator/dt ==
  Clock : Clock
  Memory1 : Memory  InitialCondition=-1
  Sum4 : Sum  Inputs=+-  InputSameDT=on  SaturateOnIntegerOverflow=on  OutDataTypeStr=Inherit: Same as first input
  Out1 : Outport  InitialOutput=0
  wires:
  Sum4/1 -> Out1/1
  Memory1/1 -> Sum4/2
  Clock/1 -> Memory1/1, Sum4/1

== system BD_PAR_SS/<vc> par/pre-TX parallel gearbox control/allow upshift?/Block NOTES1 ==
  note: This block prevents an upshift if it the engine is not on and
      | the upshift would make the motor power low enough that it
      | could not provide the required input power.  However, an upshift
      | is allowed if to stay in the current gear would put the motor
      | beyond 95% of its maximum speed.
      |
      | This block is to be used in pretransmission parallel hybrids
      | (where the engine and motor torques are combined on the
      | engine side of the transmission) ONLY.

== system BD_PAR_SS/<vc> par/pre-TX parallel gearbox control/downshift  command/load fraction ==
  In1 : Inport
  S-Function : S-Function  FunctionName=sfun_gearbox  Parameters=load, spd  SFunctionDeploymentMode=off  EnableBusSupport=off
  Out1 : Outport  InitialOutput=0
  wires:
  S-Function/1 -> Out1/1
  In1/1 -> S-Function/1

== system BD_PAR_SS/<vc> par/pre-TX parallel gearbox control/gearbox speed estimator/Block NOTES ==
  note: The requested engine speed is replaced by an estimate of the
      | engine's previous speed whenever the vehicle missed the trace
      |  by more than 1 mph on the last time step.

== system BD_PAR_SS/<vc> par/pre-TX parallel gearbox control/gearbox speed estimator/dt ==
  Clock : Clock
  Memory1 : Memory  InitialCondition=-1
  Sum4 : Sum  Inputs=+-  InputSameDT=on  SaturateOnIntegerOverflow=on  OutDataTypeStr=Inherit: Same as first input
  Out1 : Outport  InitialOutput=0
  wires:
  Sum4/1 -> Out1/1
  Memory1/1 -> Sum4/2
  Clock/1 -> Memory1/1, Sum4/1

== system BD_PAR_SS/<vc> par/pre-TX parallel gearbox control/shifting1/time since last shift ==
  in_1 : Inport
  just shifted : Subsystem
      mask Display: disp('just\nshifted')
  timer : Subsystem
      mask Display: disp('timer')
  out_1 : Outport  InitialOutput=0
  wires:
  timer/1(time) -> out_1/1
  just shifted/1(out_1) -> timer/1(trigger)
  in_1/1 -> just shifted/1(in_1)

== system BD_PAR_SS/<vc> par/pre-TX parallel gearbox control/upshift  command/load fraction ==
  In1 : Inport
  S-Function : S-Function  FunctionName=sfun_gearbox  Parameters=load, spd  SFunctionDeploymentMode=off  EnableBusSupport=off
  Out1 : Outport  InitialOutput=0
  wires:
  S-Function/1 -> Out1/1
  In1/1 -> S-Function/1

== system BD_PAR_SS/<vc> par/startStop/checkBrake/checkBrakingElapsedTime ==
  time : Inport  OutDataTypeStr=fixdt(0,16,1,0)
  braking_status : Inport  Port=2  OutDataTypeStr=fixdt(0,1,1,0)
  Constant : Constant  Value=5  OutDataTypeStr=fixdt(0,3,1,0)
  Constant1 : Constant  OutDataTypeStr=fixdt(0,1,1,0)
  Constant{2,4..6,8} (5 alike) : Constant  Value=0  OutDataTypeStr=fixdt(0,1,1,0)
  Constant3 : Constant  OutDataTypeStr=fixdt(0,1,1,0)
  Constant7 : Constant  Value=0  OutDataTypeStr=fixdt(0,16,1,0)
  Delay : Delay  DelayLength=1  InitialCondition=0
  Delay1 : Delay  DelayLength=1  InitialCondition=0
  Sum : Sum  Inputs=-|+  OutDataTypeStr=fixdt(0,16,1,0)
  Sum1 : Sum  OutDataTypeStr=fixdt(0,1,1,0)
  Sum2 : Sum  OutDataTypeStr=fixdt(0,16,1,0)
  Switch : Switch  Threshold=5  OutDataTypeStr=fixdt(0,1,1,0)
  Switch{1..2,7..8} (4 alike) : Switch  Threshold=1  OutDataTypeStr=fixdt(0,16,1,0)
  Switch3 : Switch  Threshold=1  OutDataTypeStr=fixdt(0,1,1,0)
  Switch4 : Switch  Threshold=5
  Switch5 : Switch  Threshold=1  OutDataTypeStr=fixdt(0,1,1,0)
  To Workspace1 : ToWorkspace  VariableName=ss_braking_start_time  SampleTime=-1
  To Workspace2 : ToWorkspace  VariableName=ss_braking_timer_status  SampleTime=-1
  To Workspace3 : ToWorkspace  VariableName=ss_braking_elapsed_time  SampleTime=-1
  check_braking_elapsed_time : Outport
  wires:
  Sum/1 -> Switch1/1
  time/1 -> Sum/2, Switch2/3
  Sum2/1 -> Sum/1, Switch2/1
  Constant/1 -> Switch4/1
  Constant1/1 -> Switch/1
  Constant2/1 -> Switch/3
  Switch/1 -> check_braking_elapsed_time/1
  braking_status/1 -> [braking_status]
  [braking_status] -> Switch8/2
  [braking_status] -> Switch5/2
  Switch1/1 -> Switch4/2, Switch4/3
  Constant4/1 -> Switch5/3
  [braking_status] -> Switch7/2
  Constant5/1 -> Switch7/3
  Switch3/1 -> Switch5/1
  Switch4/1 -> Switch7/1
  Switch2/1 -> Switch8/1
  Constant3/1 -> Switch3/3
  Sum1/1 -> Switch2/2, Switch1/3, Switch1/2, Switch3/1, Switch3/2
  Switch8/1 -> Delay1/1, To Workspace1/1
  Switch7/1 -> To Workspace3/1, Switch/2
  Switch5/1 -> Delay/1, To Workspace2/1
  Constant6/1 -> Sum1/1
  Constant7/1 -> Sum2/2
  Constant8/1 -> Switch8/3
  Delay/1 -> Sum1/2
  Delay1/1 -> Sum2/1

== system BD_PAR_SS/<vc> par/startStop/checkSystemLatency/checkRestartEngineElapsedTime ==
  time : Inport  OutDataTypeStr=fixdt(0,16,1,0)
  braking_status : Inport  Port=2
  Constant{8,10..12,14} (5 alike) : Constant  Value=0  OutDataTypeStr=fixdt(0,1,1,0)
  Constant13 : Constant  Value=0  OutDataTypeStr=fixdt(0,16,1,0)
  Constant6 : Constant  Value=2  OutDataTypeStr=fixdt(0,2,1,0)
  Constant7 : Constant  OutDataTypeStr=fixdt(0,1,1,0)
  Constant9 : Constant  OutDataTypeStr=fixdt(0,1,1,0)
  Delay : Delay  DelayLength=1  InitialCondition=0
  Delay1 : Delay  DelayLength=1  InitialCondition=0
  Sum1 : Sum  Inputs=-|+  OutDataTypeStr=fixdt(0,16,1,0)
  Sum2 : Sum  OutDataTypeStr=fixdt(0,1,1,0)
  Sum3 : Sum  OutDataTypeStr=fixdt(0,16,1,0)
  Switch10 : Switch  Threshold=1  OutDataTypeStr=fixdt(0,16,1,0)
  Switch11 : Switch  Threshold=1  OutDataTypeStr=fixdt(0,1,1,0)
  Switch12 : Switch  Threshold=2
  Switch13 : Switch  Threshold=1  OutDataTypeStr=fixdt(0,1,1,0)
  Switch14 : Switch  Threshold=1
  Switch15 : Switch  Threshold=1  OutDataTypeStr=fixdt(0,16,1,0)
  Switch8 : Switch  Threshold=2  OutDataTypeStr=fixdt(0,1,1,0)
  Switch9 : Switch  Threshold=1
  To Workspace1 : ToWorkspace  VariableName=ss_restart_engine_start_time  SampleTime=-1
  To Workspace2 : ToWorkspace  VariableName=ss_restart_engine_timer_status  SampleTime=-1
  To Workspace3 : ToWorkspace  VariableName=ss_restart_engine_elapsed_time  SampleTime=-1
  check_restart_engine_elapsed_time : Outport
  wires:
  Constant14/1 -> Switch15/3
  Switch13/1 -> To Workspace2/1, Delay/1
  Switch11/1 -> Switch13/1
  Sum2/1 -> Switch10/2, Switch9/3, Switch9/2, Switch11/1, Switch11/2
  Delay1/1 -> Sum3/1
  Switch14/1 -> To Workspace3/1, Switch8/2
  Constant9/1 -> Switch11/3
  [checking_status] -> Switch14/2
  Switch8/1 -> check_restart_engine_elapsed_time/1
  Switch10/1 -> Switch15/1
  Sum1/1 -> Switch9/1
  Switch15/1 -> To Workspace1/1, Delay1/1
  time/1 -> Sum1/2, Switch10/3
  Constant11/1 -> Switch14/3
  Switch12/1 -> Switch14/1
  Constant10/1 -> Switch13/3
  Constant13/1 -> Sum3/2
  braking_status/1 -> [checking_status]
  Delay/1 -> Sum2/2
  [checking_status] -> Switch15/2
  [checking_status] -> Switch13/2
  Sum3/1 -> Sum1/1, Switch10/1
  Constant8/1 -> Switch8/3
  Constant7/1 -> Switch8/1
  Constant6/1 -> Switch12/1
  Switch9/1 -> Switch12/2, Switch12/3
  Constant12/1 -> Sum2/1

== system BD_PAR_SS/electric acc loads <acc>/Electrical Accessory Loads v2 <acc>/Accessory SDO/electrical power logging ==
  In1 : Inport
  Gain : Gain  Gain=acc_elec_eff  SaturateOnIntegerOverflow=on  OutDataTypeStr=Inherit: Same as input  ParamDataTypeStr=Inherit: Same as input
  To Workspace6 : ToWorkspace  VariableName=acc_elec_pwr_in_a  SampleTime=-1
  To Workspace8 : ToWorkspace  VariableName=acc_elec_pwr_out_a  SampleTime=-1
  wires:
  Gain/1 -> To Workspace8/1
  In1/1 -> Gain/1, To Workspace6/1

== system BD_PAR_SS/electric acc loads <acc>/Electrical Accessory Loads v2 <acc>/backward model/electrical accessories (W) ==
  Electrical Accessories: Time Variable : lib_accessory/Electrical Accessories: Time Variable  SystemSampleTime=-1  VariantActivationTime=update diagram  Latency=0  AutoFrameSizeCalculation=off
  P_elec_acc : Outport
  wires:
  Electrical Accessories: Time Variable/1 -> P_elec_acc/1

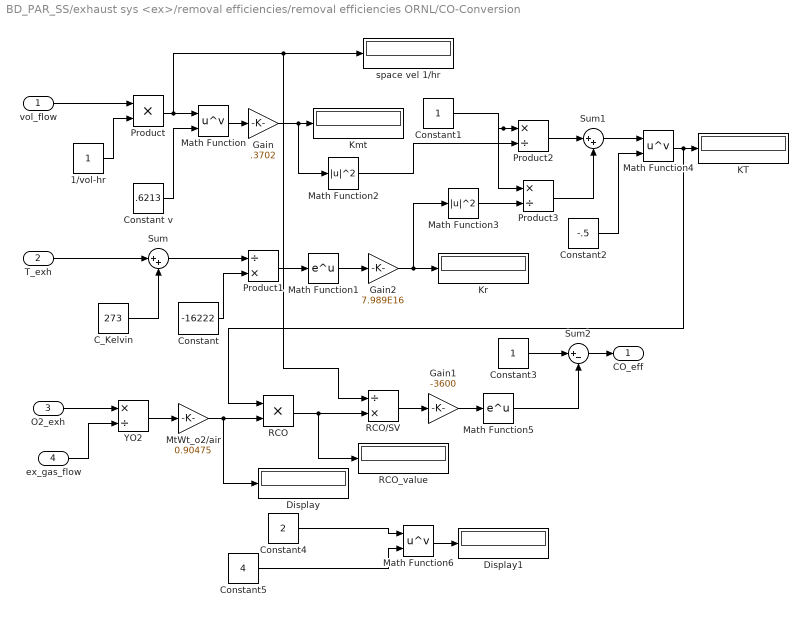
== system BD_PAR_SS/exhaust sys <ex>/removal efficiencies/removal efficiencies ORNL/CO-Conversion ==
  vol_flow : Inport
  T_exh : Inport  Port=2
  O2_exh : Inport  Port=3
  ex_gas_flow : Inport  Port=4
  1/vol-hr : Constant
  C_Kelvin : Constant  Value=273
  Constant : Constant  Value=-16222
  Constant v : Constant  Value=.6213
  Constant1 : Constant
  Constant2 : Constant  Value=-.5
  Constant3 : Constant
  Constant4 : Constant  Value=2
  Constant5 : Constant  Value=4
  Display : Display
  Display1 : Display
  Gain : Gain  Gain=.3702  SaturateOnIntegerOverflow=on
  Gain1 : Gain  Gain=-3600  SaturateOnIntegerOverflow=on
  Gain2 : Gain  Gain=7.989E16  SaturateOnIntegerOverflow=on
  KT : Display
      settings: Format=short_e
  Kmt : Display
      settings: Format=short_e
  Kr : Display
  Math Function : Math  Operator=pow  SaturateOnIntegerOverflow=on
  Math Function1 : Math  SaturateOnIntegerOverflow=on
  Math Function2 : Math  Operator=magnitude^2  SaturateOnIntegerOverflow=on
  Math Function3 : Math  Operator=magnitude^2  SaturateOnIntegerOverflow=on
  Math Function4 : Math  Operator=pow  SaturateOnIntegerOverflow=on
  Math Function5 : Math  SaturateOnIntegerOverflow=on
  Math Function6 : Math  Operator=pow  SaturateOnIntegerOverflow=on
  MtWt_o2/air : Gain  Gain=0.90475  SaturateOnIntegerOverflow=on
  Product : Product  SaturateOnIntegerOverflow=on
  Product1 : Product  Inputs=/*  SaturateOnIntegerOverflow=on
  Product2 : Product  Inputs=*/  SaturateOnIntegerOverflow=on
  Product3 : Product  Inputs=*/  SaturateOnIntegerOverflow=on
  RCO : Product  SaturateOnIntegerOverflow=on
  RCO/SV : Product  Inputs=/*  SaturateOnIntegerOverflow=on
  RCO_value : Display
  Sum : Sum  Inputs=|++  SaturateOnIntegerOverflow=on
  Sum1 : Sum  Inputs=|++  SaturateOnIntegerOverflow=on
  Sum2 : Sum  Inputs=|+-  SaturateOnIntegerOverflow=on
  YO2 : Product  Inputs=*/  SaturateOnIntegerOverflow=on
  space vel 1/hr : Display
      settings: Format=short_e
  CO_eff : Outport
  wires:
  Math Function6/1 -> Display1/1
  Constant5/1 -> Math Function6/2
  Constant4/1 -> Math Function6/1
  MtWt_o2/air/1 -> Display/1, RCO/2
  YO2/1 -> MtWt_o2/air/1
  RCO/1 -> RCO_value/1, RCO/SV/2
  Sum2/1 -> CO_eff/1
  Math Function5/1 -> Sum2/2
  Constant3/1 -> Sum2/1
  Gain1/1 -> Math Function5/1
  RCO/SV/1 -> Gain1/1
  Math Function4/1 -> RCO/1, KT/1
  ex_gas_flow/1 -> YO2/2
  O2_exh/1 -> YO2/1
  T_exh/1 -> Sum/1
  vol_flow/1 -> Product/1
  Product1/1 -> Math Function1/1
  Constant2/1 -> Math Function4/2
  Sum1/1 -> Math Function4/1
  Product3/1 -> Sum1/2
  Product2/1 -> Sum1/1
  Math Function3/1 -> Product3/2
  Math Function2/1 -> Product2/2
  Constant1/1 -> Product2/1, Product3/1
  Gain2/1 -> Math Function3/1, Kr/1
  Gain/1 -> Math Function2/1, Kmt/1
  Math Function1/1 -> Gain2/1
  Sum/1 -> Product1/1
  Constant/1 -> Product1/2
  C_Kelvin/1 -> Sum/2
  Product/1 -> RCO/SV/1, space vel 1/hr/1, Math Function/1
  Math Function/1 -> Gain/1
  Constant v/1 -> Math Function/2
  1/vol-hr/1 -> Product/2

== system BD_PAR_SS/exhaust sys <ex>/removal efficiencies/removal efficiencies ORNL/HC-Conversion ==
  vol_flow : Inport
  T_exh : Inport  Port=2
  O2_exh : Inport  Port=3
  ex_gas_flow : Inport  Port=4
  1/vol-hr : Constant
  C_Kelvin : Constant  Value=273
  Constant : Constant  Value=-10956
  Constant v : Constant  Value=.6436
  Constant2 : Constant  Value=-.1
  Constant3 : Constant
  Constant4 : Constant  Value=-2171
  Constant5 : Constant  Value=5.818
  Constant6 : Constant  Value=-10
  Gain1 : Gain  Gain=-3600  SaturateOnIntegerOverflow=on
  Gain2 : Gain  Gain=3.731E11  SaturateOnIntegerOverflow=on
  KT : Display
      settings: Format=short_e
  Kmt : Display
      settings: Format=short_e
  Kr : Display
  Math Function{,2..4} (4 alike) : Math  Operator=pow  SaturateOnIntegerOverflow=on
  Math Function1 : Math  SaturateOnIntegerOverflow=on
  Math Function5 : Math  SaturateOnIntegerOverflow=on
  Math Function6 : Math  SaturateOnIntegerOverflow=on
  MtWt_o2/air : Gain  Gain=0.90475  SaturateOnIntegerOverflow=on
  Product : Product  SaturateOnIntegerOverflow=on
  Product1 : Product  Inputs=/*  SaturateOnIntegerOverflow=on
  Product4 : Product  Inputs=*/  SaturateOnIntegerOverflow=on
  Product5 : Product  Inputs=3  SaturateOnIntegerOverflow=on
  RHC : Product  SaturateOnIntegerOverflow=on
  RHC/SV : Product  Inputs=/*  SaturateOnIntegerOverflow=on
  RHC_value : Display
  Sum : Sum  Inputs=|++  SaturateOnIntegerOverflow=on
  Sum1 : Sum  Inputs=|++  SaturateOnIntegerOverflow=on
  Sum2 : Sum  Inputs=|+-  SaturateOnIntegerOverflow=on
  YO2 : Product  Inputs=*/  SaturateOnIntegerOverflow=on
  space vel 1/hr : Display
      settings: Format=short_e
  HC_eff : Outport
  wires:
  Sum/1 -> Product4/2, Product1/1
  T_exh/1 -> Sum/1
  Math Function3/1 -> Sum1/2
  Math Function2/1 -> Sum1/1
  Constant6/1 -> Math Function3/2, Math Function2/2
  Math Function6/1 -> Product5/3
  Constant5/1 -> Product5/1
  Product4/1 -> Math Function6/1
  Constant4/1 -> Product4/1
  RHC/1 -> RHC_value/1, RHC/SV/2
  MtWt_o2/air/1 -> RHC/2
  YO2/1 -> MtWt_o2/air/1
  Sum2/1 -> HC_eff/1
  Math Function5/1 -> Sum2/2
  Constant3/1 -> Sum2/1
  Gain1/1 -> Math Function5/1
  RHC/SV/1 -> Gain1/1
  Math Function4/1 -> RHC/1, KT/1
  ex_gas_flow/1 -> YO2/2
  O2_exh/1 -> YO2/1
  vol_flow/1 -> Product/1
  Product1/1 -> Math Function1/1
  Constant2/1 -> Math Function4/2
  Sum1/1 -> Math Function4/1
  Gain2/1 -> Math Function3/1, Kr/1
  Product5/1 -> Math Function2/1, Kmt/1
  Math Function1/1 -> Gain2/1
  Constant/1 -> Product1/2
  C_Kelvin/1 -> Sum/2
  Product/1 -> RHC/SV/1, space vel 1/hr/1, Math Function/1
  Math Function/1 -> Product5/2
  Constant v/1 -> Math Function/2
  1/vol-hr/1 -> Product/2
